simulink model "Battery_Charger_Using_Boost"  (R2021a)
settings: Solver=VariableStepAuto  StartTime=0.0  StopTime=0.1  RelTol=1e-3
undefined symbols (not defined in the file): Acid, Lead
libraries: spsDiodeLib x5, spsSeriesRLCBranchLib x4, spsVoltageMeasurementLib x3, spsCurrentMeasurementLib x2, spsACVoltageSourceLib x1, spsBatteryLib x1, spsLinearTransformerLib x1, spsMosfetLib x1, pid_lib x1, spsPWMGeneratorDCDCLib x1, eePowerMeasurement x1, spspowerguiLib x1
settings Model: Creator=gupta  LastModifiedBy=gupta

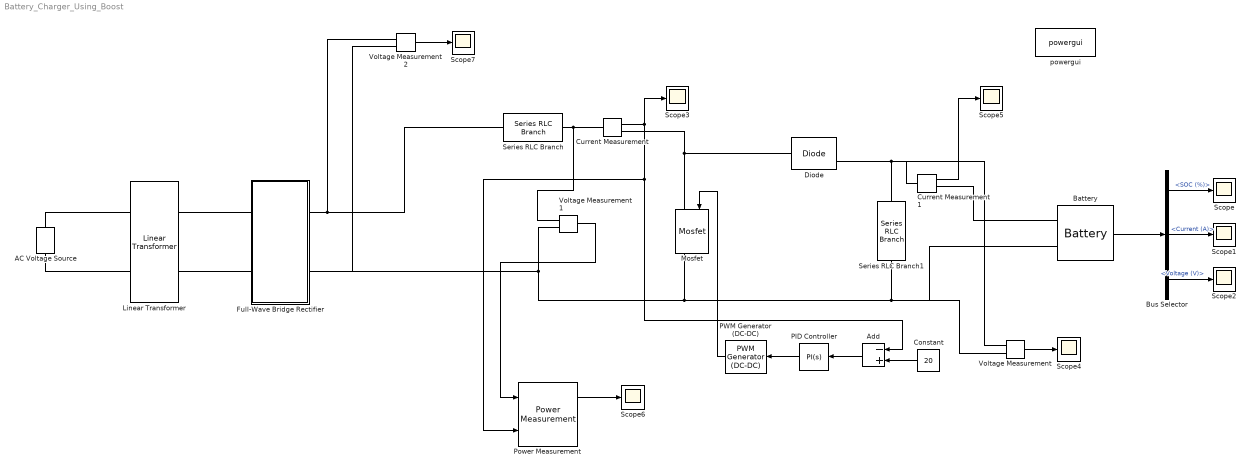
== system Battery_Charger_Using_Boost ==
  AC Voltage Source : spsACVoltageSourceLib/AC Voltage Source  Amplitude=325.269  Phase=0  Frequency=50  SampleTime=5e-6  Measurements=None  BusType=swing  Pref=10e3  Qref=0  Qmin=-inf  Qmax=+inf
  Add : Sum  Inputs=-+
  Battery : spsBatteryLib/Battery  BatType=Lead-Acid  ShowTempParam=off  ThermalPreset=no  ShowAgeParam=off  NomV=48  NomQ=28  SOC=45  Batt_Tr=5e-6  PresetModel=on  MaxQ=29.1667  MinV=36  FullV=52.2632  Dis_rate=5.6  R=0.017143  Normal_OP=8.6878  expZone="[48.8684    0.0933333]"  current=[6.5 13 32.5]  Units=Time  Tci=20  NomT=20  T2=-30  MaxQ2=4.8  FullV2=7.1  Normal_OP2=5.655  expZone2="[6.58           1]"  Rca=0.6  ti=2000  Dp=0  Neq0=0  Tsim=1e6  Ta1=25  Qeol=5.4*0.9  Reol=0.013333*1.2  Char_age=[2.3478, 3]  Dis_age=[2.3478, 10]  N1=1500  N2=10500  N3=1000  N4=1400  Ta2=45  N5=950
  Bus Selector : BusSelector  OutputSignals=SOC (%),Current (A),Voltage (V)
  Constant : Constant  Value=20
  Current Measurement : spsCurrentMeasurementLib/Current Measurement  PhasorSimulation=off  OutputType=Complex  PSBequivalent=0
  Current Measurement1 : spsCurrentMeasurementLib/Current Measurement  PhasorSimulation=off  OutputType=Complex  PSBequivalent=0
  Diode : spsDiodeLib/Diode  Ron=0.001  Lon=0  Vf=0.8  IC=0  UseSnubber=0  Rs=500  Cs=250e-9  Measurements=on
  Full-Wave Bridge Rectifier : Subsystem
  Linear Transformer : spsLinearTransformerLib/Linear Transformer  UNITS=SI  NominalPower=[ 1e3 50 ]  winding1=[10 0 0]  winding2=[1 0 0]  ThreeWindings=off  winding3=[3.15e+05 1.9845e+05 25267]  RmLm=[Inf Inf]  Measurements=None  DataType=on
  Mosfet : spsMosfetLib/Mosfet  Ron=0.001  Lon=0  Rd=0.001  Vfd=0  IC=0  Rs=1e5  Cs=inf  Measurements=on
  PID Controller : pid_lib/PID Controller  Controller=PI  Form=Parallel  TimeDomain=Continuous-time  UseExternalTs=off  SampleTime=-1  IntegratorMethod=Forward Euler  FilterMethod=Forward Euler  ControllerParametersSource=internal  P=10  I=1  D=0  UseFilter=on  N=100  TunerSelectOption=Transfer Function Based (PID Tuner App)  InitialConditionSource=internal  InitialConditionForIntegrator=0  InitialConditionForFilter=0  DifferentiatorICPrevScaledInput=0  ExternalReset=none  TrackingMode=off  Kt=1  LimitOutput=off  SatLimitsSource=internal  UpperSaturationLimit=inf  LowerSaturationLimit=-inf  LinearizeAsGain=on  AntiWindupMode=none  Kb=1  POutMin=[]  POutMax=[]  IOutMin=[]  IOutMax=[]  DOutMin=[]  DOutMax=[]  NOutMin=[]  NOutMax=[]  SumOutMin=[]  SumOutMax=[]  SaturationOutMin=[]  SaturationOutMax=[]  PParamMin=[]  PParamMax=[]  IParamMin=[]  IParamMax=[]  DParamMin=[]  DParamMax=[]  NParamMin=[]  NParamMax=[]  KbParamMin=[]  KbParamMax=[]  KtParamMin=[]  KtParamMax=[]  KbOutMin=[]  KbOutMax=[]  KtOutMin=[]  KtOutMax=[]  IntegratorOutMin=[]  IntegratorOutMax=[]  FilterOutMin=[]  FilterOutMax=[]  SumI1OutMin=[]  SumI1OutMax=[]  SumI2OutMin=[]  SumI2OutMax=[]  SumI3OutMin=[]  SumI3OutMax=[]  SumI4OutMin=[]  SumI4OutMax=[]  SumDOutMin=[]  SumDOutMax=[]  DifferentiatorOutMin=[]  DifferentiatorOutMax=[]  FilterDiffOutCoefMin=[]  FilterDiffOutCoefMax=[]  ReciprocalOutMin=[]  ReciprocalOutMax=[]  SumDenOutMin=[]  SumDenOutMax=[]  SumNumOutMin=[]  SumNumOutMax=[]  DivideOutMin=[]  DivideOutMax=[]  UdiffTsProdOutMin=[]  UdiffTsProdOutMax=[]  NTsProdOutMin=[]  NTsProdOutMax=[]  UintegralTsProdOutMin=[]  UintegralTsProdOutMax=[]  UngainTsProdOutMin=[]  UngainTsProdOutMax=[]  IntegratorContinuousStateAttributes=''  IntegratorStateMustResolveToSignalObject=off  IntegratorRTWStateStorageClass=Auto  FilterContinuousStateAttributes=''  FilterStateMustResolveToSignalObject=off  FilterRTWStateStorageClass=Auto  ParallelPVariant=InternalParameters  IdealPVariant=Disabled  IVariant=InternalParameters  DVariant=Disabled  IntegratorVariant=Continuous  SatVariant=Disabled  AWVariant=Passthrough  PCopyVariant=Disabled  TRVariant=Disabled  FdbkBlocksVariant=Forward  IdealPFdbkVariant=Disabled  SatFdbkVariant=Disabled  DerivativeFilterVariant=Disabled  NVariant=Disabled  NCopyVariant=Disabled_SignalSpec  FilterICVariant=Disabled  IntegratorICVariant=InternalICs  ExternalResetVariant=Disabled  TRSumVariant=Passthrough  SumFdbkVariant=Disabled  SumVariant=Sum_PI  TsampFilterVariant=InternalTs  TsampNgainVariant=Passthrough  TsampIntegralVariant=Passthrough  ExternalSaturationOutDataTypeStr=Inherit: Same as second input
  PWM Generator (DC-DC) : spsPWMGeneratorDCDCLib/PWM Generator (DC-DC)  Fsw=30000  Ts=5e-6
  Power Measurement : eePowerMeasurement/Power Measurement  LabelModeActiveChoice=Discrete  F=50  K=[0 1 2 3]  Ts=5e-6
      settings: SourceProductBaseCode=PS
  Scope{,1..7} (8 alike) : Scope
  Series RLC Branch : spsSeriesRLCBranchLib/Series RLC Branch  LConnTagsString=__new0  RConnTagsString=__new0  BranchType=L  Resistance=1  Inductance=1.309e-3  SetiL0=off  InitialCurrent=0  Capacitance=1e-6  Setx0=off  InitialVoltage=0  Measurements=None
  Series RLC Branch1 : spsSeriesRLCBranchLib/Series RLC Branch  LConnTagsString=__new0  RConnTagsString=__new0  BranchType=C  Resistance=1  Inductance=1e-3  SetiL0=off  InitialCurrent=0  Capacitance=138.138e-6  Setx0=off  InitialVoltage=0  Measurements=None
  Voltage Measurement : spsVoltageMeasurementLib/Voltage Measurement  PhasorSimulation=off  OutputType=Complex  PSBequivalent=0
  Voltage Measurement1 : spsVoltageMeasurementLib/Voltage Measurement  PhasorSimulation=off  OutputType=Complex  PSBequivalent=0
  Voltage Measurement2 : spsVoltageMeasurementLib/Voltage Measurement  PhasorSimulation=off  OutputType=Complex  PSBequivalent=0
  powergui : spspowerguiLib/powergui  Priority=1  SimulationMode=Continuous  SampleTime=50e-6  frequency=60  Iterations=50  frequencyindice=0  Pbase=100e6  ErrMax=1e-4  UnitsV=kV  UnitsW=MW  buscounter=0  FunctionMessages=off  echomessages=off  EnableUseOfTLC=off  CurrentSourceSwitches=off  DisableSnubberDevices=off  DisableRonSwitches=off  DisableVfSwitches=off  DisplayEquations=off  AutomaticDiscreteSolvers=off  SolverType=Tustin/Backward Euler (TBE)  Interpol=off  ExternalGateDelay=off  methode=off  Ts=100  x0status=blocks  SPID=on  SwTol=0  HookPort=off  NonlinearTolerance=1e-4  nMaxIteration=100  ContinueOnMaxIteration=off  RestoreLinks=warning  ResistiveCurrentMeasurement=off  Frange=[0:2:500]  Ylog=off  Xlog=on  ShowGrid=off  save=off  variable=ZData  structure=0  ZoomFFT=off  StartTime=0.0  cycles=1  DisplayStyle=1  fundamental=60  FreqAxis=off  MaxFrequency=1000  frequencyindicesteady=1  RmsSteady=1  display=off
  wires:
  Battery/1 -> Bus Selector/1
  Bus Selector/1 -> Scope/1  "<SOC (%)>"
  Bus Selector/2 -> Scope1/1  "<Current (A)>"
  Bus Selector/3 -> Scope2/1  "<Voltage (V)>"
  Current Measurement/1 -> Scope3/1, Power Measurement/2, Add/1
  Voltage Measurement/1 -> Scope4/1
  PWM Generator (DC-DC)/1 -> Mosfet/1
  PID Controller/1 -> PWM Generator (DC-DC)/1
  Add/1 -> PID Controller/1
  Constant/1 -> Add/2
  Current Measurement1/1 -> Scope5/1
  Voltage Measurement1/1 -> Power Measurement/1
  Power Measurement/1 -> Scope6/1
  Voltage Measurement2/1 -> Scope7/1
  connections:
  Mosfet/LConn1 -- Current Measurement/RConn1 -- Diode/LConn1
  Series RLC Branch1/LConn1 -- Voltage Measurement/LConn1 -- Current Measurement1/LConn1 -- Diode/RConn1
  Current Measurement/LConn1 -- Voltage Measurement1/LConn1 -- Series RLC Branch/RConn1
  Current Measurement1/RConn1 -- Battery/LConn1
  Linear Transformer/LConn1 -- AC Voltage Source/RConn1
  Linear Transformer/LConn2 -- AC Voltage Source/LConn1
  Series RLC Branch1/RConn1 -- Battery/LConn2 -- Voltage Measurement/LConn2 -- Full-Wave Bridge Rectifier/RConn2 -- Voltage Measurement2/LConn2 -- Voltage Measurement1/LConn2 -- Mosfet/RConn1
  Linear Transformer/RConn1 -- Full-Wave Bridge Rectifier/LConn1
  Linear Transformer/RConn2 -- Full-Wave Bridge Rectifier/LConn2
  Full-Wave Bridge Rectifier/RConn1 -- Voltage Measurement2/LConn1 -- Series RLC Branch/LConn1

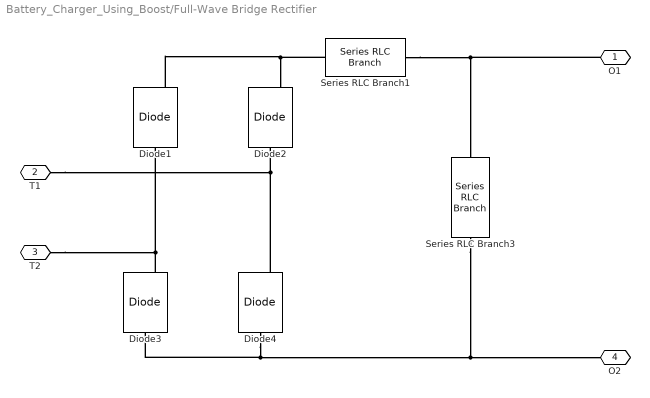
== system Battery_Charger_Using_Boost/Full-Wave Bridge Rectifier ==
  Diode{1..4} (4 alike) : spsDiodeLib/Diode  Ron=0.001  Lon=0  Vf=0.8  IC=0  UseSnubber=0  Rs=500  Cs=250e-9  Measurements=on
  Series RLC Branch1 : spsSeriesRLCBranchLib/Series RLC Branch  LConnTagsString=__new0  RConnTagsString=__new0  BranchType=L  Resistance=1  Inductance=1e-3  SetiL0=off  InitialCurrent=0  Capacitance=1e-6  Setx0=off  InitialVoltage=0  Measurements=None
  Series RLC Branch3 : spsSeriesRLCBranchLib/Series RLC Branch  LConnTagsString=__new0  RConnTagsString=__new0  BranchType=C  Resistance=1  Inductance=1e-3  SetiL0=off  InitialCurrent=0  Capacitance=6000e-6  Setx0=off  InitialVoltage=0  Measurements=None
  O1 : PMIOPort  Side=Right
  T1 : PMIOPort  Port=2  Side=Left
  T2 : PMIOPort  Port=3  Side=Left
  O2 : PMIOPort  Port=4  Side=Right
  connections:
  Diode3/RConn1 -- T2/RConn1 -- Diode1/LConn1
  Diode4/RConn1 -- T1/RConn1 -- Diode2/LConn1
  Diode1/RConn1 -- Series RLC Branch1/LConn1 -- Diode2/RConn1
  Diode4/LConn1 -- O2/RConn1 -- Series RLC Branch3/RConn1 -- Diode3/LConn1
  O1/RConn1 -- Series RLC Branch1/RConn1 -- Series RLC Branch3/LConn1
